simulink model "Rectifier_3"  (R2022a)
settings: Solver=VariableStepAuto  StartTime=0.0  StopTime=2  RelTol=1e-3
model workspace (MAT data in the model file):
  reset = 0
undefined symbols (not defined in the file): DiscIntNeverNeededParam
libraries: spsSeriesRLCBranchLib x38, spsDiodeLib x14, spsCurrentMeasurementLib x12, spsIGBTDiodeLib x8, spsIdealSwitchLib x7, spsMosfetLib x6, spsVoltageMeasurementLib x6, slpidlib x5, spsLinearTransformerLib x4, spsACVoltageSourceLib x3, spsabctodq0Lib x2, simulink x2
settings Model: Creator=zhang  LastModifiedBy=zhang
settings DebuggingCC: UnconnectedInputMsg=warning  UnconnectedOutputMsg=warning  UnconnectedLineMsg=warning
settings RTWCC: DLArmComputeVersion=19.05

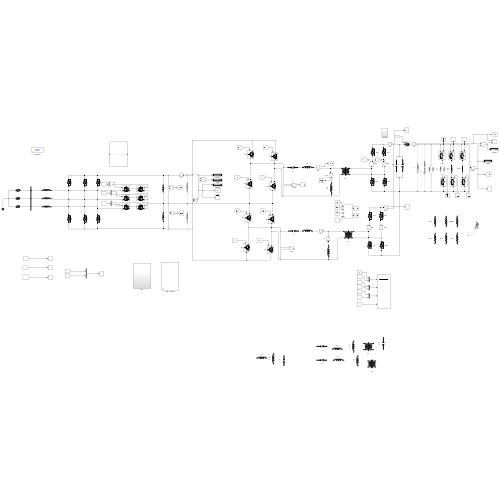
[thumbnail: Simulink's stored preview of the top-level diagram]
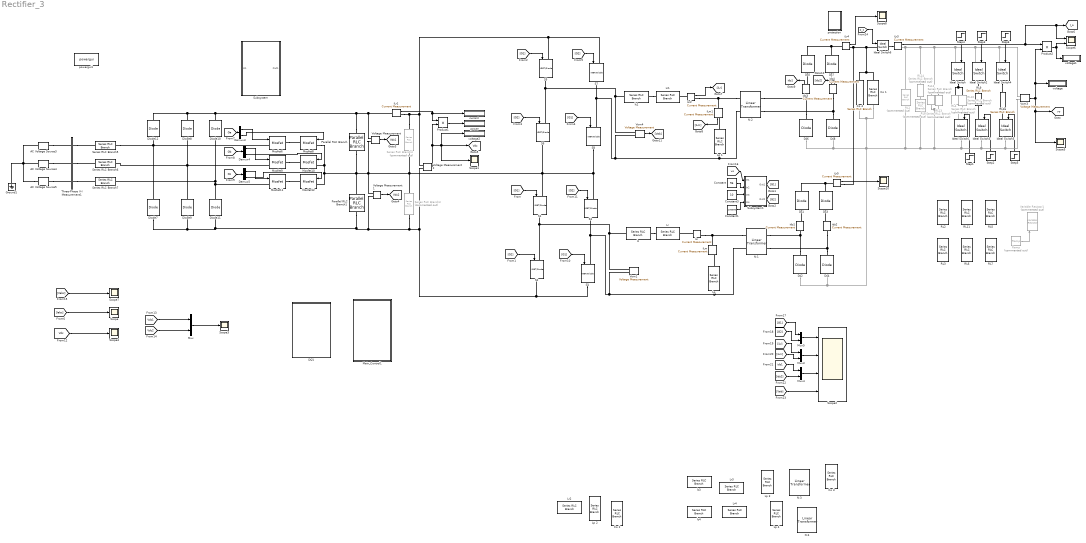
== system Rectifier_3 ==
  " protection" : Subsystem
  AC Voltage Source3 : spsACVoltageSourceLib/AC Voltage Source  Amplitude=311  Phase=0  Frequency=50  SampleTime=0  Measurements=None  BusType=swing  Pref=10e3  Qref=0  Qmin=-inf  Qmax=+inf
  AC Voltage Source4 : spsACVoltageSourceLib/AC Voltage Source  Amplitude=311  Phase=240  Frequency=50  SampleTime=0  Measurements=None  BusType=swing  Pref=10e3  Qref=0  Qmin=-inf  Qmax=+inf
  AC Voltage Source5 : spsACVoltageSourceLib/AC Voltage Source  Amplitude=311  Phase=120  Frequency=50  SampleTime=0  Measurements=None  BusType=swing  Pref=10e3  Qref=0  Qmin=-inf  Qmax=+inf
  Co 1 : spsSeriesRLCBranchLib/Series RLC Branch  LConnTagsString=__new0  RConnTagsString=__new0  BranchType=C  Resistance=1e-3  Inductance=1e-3  SetiL0=off  InitialCurrent=0  Capacitance=10e-3  Setx0=off  InitialVoltage=96  Measurements=None
  Co 2 : spsSeriesRLCBranchLib/Series RLC Branch  LConnTagsString=__new0  RConnTagsString=__new0  BranchType=C  Resistance=1  Inductance=1e-3  SetiL0=off  InitialCurrent=0  Capacitance=660e-6  Setx0=off  InitialVoltage=0  Measurements=None
  Co 3 : spsSeriesRLCBranchLib/Series RLC Branch  LConnTagsString=__new0  RConnTagsString=__new0  BranchType=C  Resistance=1  Inductance=1e-3  SetiL0=off  InitialCurrent=0  Capacitance=2100e-6  Setx0=off  InitialVoltage=0  Measurements=None
  Co 4 : spsSeriesRLCBranchLib/Series RLC Branch  LConnTagsString=__new0  RConnTagsString=__new0  BranchType=C  Resistance=1e-3  Inductance=1e-3  SetiL0=off  InitialCurrent=0  Capacitance=4e-3  Setx0=off  InitialVoltage=96  Measurements=None
  Constant : Constant  Value=96
  Constant1 : Constant  Value=100000
  Constant3 : Constant  Value=10
  DQ1 : Subsystem
  Demux3 : Demux  Outputs=2
  Demux4 : Demux  Outputs=2
  Demux5 : Demux  Outputs=2
  Diode{7..12} (6 alike) : spsDiodeLib/Diode  Ron=0.001  Lon=0  Vf=0.8  IC=0  UseSnubber=off  Rs=1e5  Cs=250e-9  Measurements=off
  Ds{1..8} (8 alike) : spsDiodeLib/Diode  Ron=0.001  Lon=0  Vf=0.8  IC=0  UseSnubber=0  Rs=500  Cs=250e-9  Measurements=off
  Ground1 : spsGroundLib/Ground  LConnTagsString=a
  Ideal Switch{,1..6} (7 alike) : spsIdealSwitchLib/Ideal Switch  Ron=0.001  Lon=0  IC=0  Rs=1e5  Cs=inf  Measurements=off
  "Lp " : spsSeriesRLCBranchLib/Series RLC Branch  LConnTagsString=__new0  RConnTagsString=__new0  BranchType=L  Resistance=1  Inductance=175e-6  SetiL0=off  InitialCurrent=0  Capacitance=1e-6  Setx0=off  InitialVoltage=0  Measurements=None
  Lp 1 : spsSeriesRLCBranchLib/Series RLC Branch  LConnTagsString=__new0  RConnTagsString=__new0  BranchType=L  Resistance=1  Inductance=175e-6  SetiL0=off  InitialCurrent=0  Capacitance=1e-6  Setx0=off  InitialVoltage=0  Measurements=None
  Lp 2 : spsSeriesRLCBranchLib/Series RLC Branch  LConnTagsString=__new0  RConnTagsString=__new0  BranchType=L  Resistance=1  Inductance=180.2e-6  SetiL0=off  InitialCurrent=0  Capacitance=1e-6  Setx0=off  InitialVoltage=0  Measurements=None
  Lp 3 : spsSeriesRLCBranchLib/Series RLC Branch  LConnTagsString=__new0  RConnTagsString=__new0  BranchType=L  Resistance=1  Inductance=79.6e-6  SetiL0=off  InitialCurrent=0  Capacitance=1e-6  Setx0=off  InitialVoltage=0  Measurements=None
  Lp 4 : spsSeriesRLCBranchLib/Series RLC Branch  LConnTagsString=__new0  RConnTagsString=__new0  BranchType=L  Resistance=1  Inductance=66.6e-6  SetiL0=off  InitialCurrent=0  Capacitance=1e-6  Setx0=off  InitialVoltage=0  Measurements=None
  Lr : spsSeriesRLCBranchLib/Series RLC Branch  LConnTagsString=__new0  RConnTagsString=__new0  BranchType=L  Resistance=1  Inductance=36e-6  SetiL0=off  InitialCurrent=0  Capacitance=1e-6  Setx0=off  InitialVoltage=0  Measurements=None
  Lr1 : spsSeriesRLCBranchLib/Series RLC Branch  LConnTagsString=__new0  RConnTagsString=__new0  BranchType=L  Resistance=1  Inductance=36e-6  SetiL0=off  InitialCurrent=0  Capacitance=1e-6  Setx0=off  InitialVoltage=0  Measurements=None
  Lr2 : spsSeriesRLCBranchLib/Series RLC Branch  LConnTagsString=__new0  RConnTagsString=__new0  BranchType=L  Resistance=1  Inductance=20.2e-6  SetiL0=off  InitialCurrent=0  Capacitance=1e-6  Setx0=off  InitialVoltage=0  Measurements=None
  Lr3 : spsSeriesRLCBranchLib/Series RLC Branch  LConnTagsString=__new0  RConnTagsString=__new0  BranchType=L  Resistance=1  Inductance=11.8e-6  SetiL0=off  InitialCurrent=0  Capacitance=1e-6  Setx0=off  InitialVoltage=0  Measurements=None
  Lr4 : spsSeriesRLCBranchLib/Series RLC Branch  LConnTagsString=__new0  RConnTagsString=__new0  BranchType=L  Resistance=1  Inductance=16.8e-6  SetiL0=off  InitialCurrent=0  Capacitance=1e-6  Setx0=off  InitialVoltage=0  Measurements=None
  Main_Control1 : Subsystem  mask{Vref=800, Fs=20000, Kp_v=0.53, Ki_v=0.00025, Kp_i=11, Ki_i=0.3, limit1=40, limit2=450, Kp_vb=0.5, Ki_vb=0.00001, k3=0.245}
      mask prompts: Vref "DC_voltage"; Kp_vb "VoltageBalance_Kp"; Ki_vb "VoltageBalance_Ki"
  Mosfet{6,8..12} (6 alike) : spsMosfetLib/Mosfet  Ron=0.1  Lon=0  Rd=0.01  Vfd=0  IC=0  Rs=1e5  Cs=inf  Measurements=off
  Mux{,3..5} (4 alike) : Mux  Inputs=2
  N:1 : spsLinearTransformerLib/Linear Transformer  UNITS=SI  NominalPower=[ 3e3 20000 ]  winding1=[40 0 0]  winding2=[8 0 0]  ThreeWindings=off  winding3=[355 0 0]  RmLm=[2.3349e+09 0]  Measurements=None  DataType=on
  N:2 : spsLinearTransformerLib/Linear Transformer  UNITS=SI  NominalPower=[ 3e3 20000 ]  winding1=[40 0 0]  winding2=[8 0 0]  ThreeWindings=off  winding3=[355 0 0]  RmLm=[2.3349e+09 0]  Measurements=None  DataType=on
  N:3 : spsLinearTransformerLib/Linear Transformer  UNITS=SI  NominalPower=[ 3e3 20000 ]  winding1=[400 0 0]  winding2=[90 0 0]  ThreeWindings=off  winding3=[355 0 0]  RmLm=[2.3349e+09 0]  Measurements=None  DataType=on
  N:4 : spsLinearTransformerLib/Linear Transformer  UNITS=SI  NominalPower=[ 3e3 20000 ]  winding1=[400 0 0]  winding2=[80 0 0]  ThreeWindings=off  winding3=[355 0 0]  RmLm=[2.3349e+09 0]  Measurements=None  DataType=on
  Parallel RLC Branch : spsParallelRLCBranchLib/Parallel RLC Branch  LConnTagsString=a  RConnTagsString=__new0  BranchType=C  Resistance=51e3  Inductance=1e-3  SetiL0=off  InitialCurrent=0  Capacitance=2e-3  Setx0=on  InitialVoltage=250  Measurements=None
  Parallel RLC Branch1 : spsParallelRLCBranchLib/Parallel RLC Branch  LConnTagsString=a  RConnTagsString=__new0  BranchType=C  Resistance=51e3  Inductance=1e-3  SetiL0=off  InitialCurrent=0  Capacitance=2e-3  Setx0=on  InitialVoltage=250  Measurements=None
  Product1 : Product
  Product2 : Product
  RL{1,4,12,14} (4 alike) : spsSeriesRLCBranchLib/Series RLC Branch  Commented=on  LConnTagsString=__new0  RConnTagsString=__new0  BranchType=R  Resistance=0.9216  Inductance=1e-3  SetiL0=off  InitialCurrent=0  Capacitance=3000e-6  Setx0=off  InitialVoltage=0  Measurements=None
  RL10 : spsSeriesRLCBranchLib/Series RLC Branch  Commented=on  LConnTagsString=__new0  RConnTagsString=__new0  BranchType=C  Resistance=0.9216  Inductance=1e-3  SetiL0=off  InitialCurrent=0  Capacitance=3000e-6  Setx0=off  InitialVoltage=0  Measurements=None
  RL11 : spsSeriesRLCBranchLib/Series RLC Branch  LConnTagsString=__new0  RConnTagsString=__new0  BranchType=R  Resistance=1.2288  Inductance=1e-3  SetiL0=off  InitialCurrent=0  Capacitance=2200e-6  Setx0=off  InitialVoltage=0  Measurements=None
  RL13 : spsSeriesRLCBranchLib/Series RLC Branch  Commented=on  LConnTagsString=__new0  RConnTagsString=__new0  BranchType=C  Resistance=0.9216  Inductance=1e-3  SetiL0=off  InitialCurrent=0  Capacitance=3000e-6  Setx0=off  InitialVoltage=0  Measurements=None
  RL16 : spsSeriesRLCBranchLib/Series RLC Branch  LConnTagsString=__new0  RConnTagsString=__new0  BranchType=R  Resistance=3  Inductance=1e-3  SetiL0=off  InitialCurrent=0  Capacitance=3000e-6  Setx0=off  InitialVoltage=0  Measurements=None
  RL2 : spsSeriesRLCBranchLib/Series RLC Branch  LConnTagsString=__new0  RConnTagsString=__new0  BranchType=R  Resistance=1.8432  Inductance=1e-3  SetiL0=off  InitialCurrent=0  Capacitance=2200e-6  Setx0=off  InitialVoltage=0  Measurements=None
  RL3 : spsSeriesRLCBranchLib/Series RLC Branch  LConnTagsString=__new0  RConnTagsString=__new0  BranchType=R  Resistance=3.6864  Inductance=1e-3  SetiL0=off  InitialCurrent=0  Capacitance=2200e-6  Setx0=off  InitialVoltage=0  Measurements=None
  RL5 : spsSeriesRLCBranchLib/Series RLC Branch  LConnTagsString=__new0  RConnTagsString=__new0  BranchType=R  Resistance=1.8432  Inductance=1e-3  SetiL0=off  InitialCurrent=0  Capacitance=2200e-6  Setx0=off  InitialVoltage=0  Measurements=None
  RL6 : spsSeriesRLCBranchLib/Series RLC Branch  LConnTagsString=__new0  RConnTagsString=__new0  BranchType=R  Resistance=1.8432  Inductance=1e-3  SetiL0=off  InitialCurrent=0  Capacitance=2200e-6  Setx0=off  InitialVoltage=0  Measurements=None
  RL7 : spsSeriesRLCBranchLib/Series RLC Branch  LConnTagsString=__new0  RConnTagsString=__new0  BranchType=R  Resistance=3.6864  Inductance=1e-3  SetiL0=off  InitialCurrent=0  Capacitance=2200e-6  Setx0=off  InitialVoltage=0  Measurements=None
  RL8 : spsSeriesRLCBranchLib/Series RLC Branch  Commented=on  LConnTagsString=__new0  RConnTagsString=__new0  BranchType=C  Resistance=0.9216  Inductance=1e-3  SetiL0=off  InitialCurrent=0  Capacitance=3000e-6  Setx0=off  InitialVoltage=0  Measurements=None
  RL9 : spsSeriesRLCBranchLib/Series RLC Branch  LConnTagsString=__new0  RConnTagsString=__new0  BranchType=R  Resistance=0.9216  Inductance=1e-3  SetiL0=off  InitialCurrent=0  Capacitance=3000e-6  Setx0=off  InitialVoltage=0  Measurements=None
  Ramp : simulink/Sources/Ramp  Commented=on  slope=9600000  start=0  InitialOutput=0
  S{1..8} (8 alike) : spsIGBTDiodeLib/IGBT//Diode  Ron=1e-3  Rs=1e5  Cs=250e-9  Measurements=off
  Scope{,1,3..5,7..8,10} (8 alike) : Scope
  Scope2 : Scope  NumInputPorts=4
  Scope6 : Scope  NumInputPorts=2
  Series RLC Branch3 : spsSeriesRLCBranchLib/Series RLC Branch  Commented=on  LConnTagsString=__new0  RConnTagsString=__new0  BranchType=R  Resistance=32  Inductance=2e-3  SetiL0=off  InitialCurrent=0  Capacitance=1e-6  Setx0=off  InitialVoltage=0  Measurements=None
  Series RLC Branch4 : spsSeriesRLCBranchLib/Series RLC Branch  Commented=on  LConnTagsString=__new0  RConnTagsString=__new0  BranchType=R  Resistance=32  Inductance=2e-3  SetiL0=off  InitialCurrent=0  Capacitance=1e-6  Setx0=off  InitialVoltage=0  Measurements=None
  Series RLC Branch5 : spsSeriesRLCBranchLib/Series RLC Branch  LConnTagsString=__new0  RConnTagsString=__new0  BranchType=L  Resistance=20  Inductance=2.5e-3  SetiL0=off  InitialCurrent=0  Capacitance=1e-6  Setx0=off  InitialVoltage=0  Measurements=None
  Series RLC Branch6 : spsSeriesRLCBranchLib/Series RLC Branch  LConnTagsString=__new0  RConnTagsString=__new0  BranchType=L  Resistance=20  Inductance=2.5e-3  SetiL0=off  InitialCurrent=0  Capacitance=1e-6  Setx0=off  InitialVoltage=0  Measurements=None
  Series RLC Branch7 : spsSeriesRLCBranchLib/Series RLC Branch  LConnTagsString=__new0  RConnTagsString=__new0  BranchType=L  Resistance=20  Inductance=2.5e-3  SetiL0=off  InitialCurrent=0  Capacitance=1e-6  Setx0=off  InitialVoltage=0  Measurements=None
  Step1 : Step  Time=0.4  Before=1  After=0  SampleTime=0
  Step2 : Step  Time=0.5  Before=1  After=0  SampleTime=0
  Step3 : Step  Time=0  SampleTime=0
  Step4 : Step  Time=0.2  SampleTime=0
  Step5 : Step  Time=1.5  Before=1  After=0  SampleTime=0
  Step6 : Step  SampleTime=0
  Subsystem : Subsystem
      settings: OpenFcn="open(\"C:\\Users\\zhang\\Desktop\\仿真\\pros\""
  Subsystem1 : Subsystem  mask{P=35000, I=5000}
      mask DialogControl ParameterGroupVar Prompt: 参数
  Three-Phase V-I Measurement1 : spsThreePhaseVIMeasurementLib/Three-Phase V-I Measurement  VoltageMeasurement=phase-to-ground  SetLabelV=on  LabelV=Vabc  Vpu=off  VpuLL=off  CurrentMeasurement=yes  SetLabelI=on  LabelI=Iabc  Ipu=off  Pbase=100e6  Vbase=500e3  OutputType=Complex  PhasorSimulation=off  PSBequivalent=0
  Variable Resistor1 : spsVariableResistorLib/Variable Resistor  Commented=on  Rabsmin=1.8432
      settings: SourceProductBaseCode=PS
  Voltage Measurement : spsVoltageMeasurementLib/Voltage Measurement  PhasorSimulation=off  OutputType=Complex  PSBequivalent=0
  Voltage Measurement1 : spsVoltageMeasurementLib/Voltage Measurement  PhasorSimulation=off  OutputType=Complex  PSBequivalent=0
  Voltage Measurement2 : spsVoltageMeasurementLib/Voltage Measurement  PhasorSimulation=off  OutputType=Complex  PSBequivalent=0
  Vom1 : spsVoltageMeasurementLib/Voltage Measurement  PhasorSimulation=off  OutputType=Complex  PSBequivalent=0
  Vom3 : spsVoltageMeasurementLib/Voltage Measurement  PhasorSimulation=off  OutputType=Complex  PSBequivalent=0
  Vom4 : spsVoltageMeasurementLib/Voltage Measurement  PhasorSimulation=off  OutputType=Complex  PSBequivalent=0
  current : Display
  iLm : spsCurrentMeasurementLib/Current Measurement  PhasorSimulation=off  OutputType=Complex  PSBequivalent=0
  iLm1 : spsCurrentMeasurementLib/Current Measurement  PhasorSimulation=off  OutputType=Complex  PSBequivalent=0
  iLr{,1..5} (6 alike) : spsCurrentMeasurementLib/Current Measurement  PhasorSimulation=off  OutputType=Complex  PSBequivalent=0
  ids{1..4} (4 alike) : spsCurrentMeasurementLib/Current Measurement  PhasorSimulation=off  OutputType=Complex  PSBequivalent=0
  lc : spsSeriesRLCBranchLib/Series RLC Branch  LConnTagsString=__new0  RConnTagsString=__new0  BranchType=C  Resistance=1  Inductance=1e-3  SetiL0=off  InitialCurrent=0  Capacitance=89.5e-9  Setx0=off  InitialVoltage=0  Measurements=None
  lc1 : spsSeriesRLCBranchLib/Series RLC Branch  LConnTagsString=__new0  RConnTagsString=__new0  BranchType=C  Resistance=1  Inductance=1e-3  SetiL0=off  InitialCurrent=0  Capacitance=89.5e-9  Setx0=off  InitialVoltage=0  Measurements=None
  lc3 : spsSeriesRLCBranchLib/Series RLC Branch  LConnTagsString=__new0  RConnTagsString=__new0  BranchType=C  Resistance=1  Inductance=1e-3  SetiL0=off  InitialCurrent=0  Capacitance=100.4e-9  Setx0=off  InitialVoltage=0  Measurements=None
  lc4 : spsSeriesRLCBranchLib/Series RLC Branch  LConnTagsString=__new0  RConnTagsString=__new0  BranchType=C  Resistance=1  Inductance=1e-3  SetiL0=off  InitialCurrent=0  Capacitance=200.4e-9  Setx0=off  InitialVoltage=0  Measurements=None
  power : Display
  powergui1 : spspowerguiLib/powergui  Priority=1  SimulationMode=Discrete  SampleTime=1e-6  frequency=60  Iterations=50  frequencyindice=0  Pbase=100e6  ErrMax=1e-4  UnitsV=kV  UnitsW=MW  buscounter=0  FunctionMessages=off  echomessages=off  EnableUseOfTLC=off  CurrentSourceSwitches=off  DisableSnubberDevices=off  DisableRonSwitches=off  DisableVfSwitches=off  DisplayEquations=off  AutomaticDiscreteSolvers=off  SolverType=Tustin/Backward Euler (TBE)  Interpol=off  ExternalGateDelay=off  methode=off  Ts=100  x0status=blocks  SPID=on  SwTol=0  HookPort=off  NonlinearTolerance=1e-4  nMaxIteration=100  ContinueOnMaxIteration=off  RestoreLinks=warning  ResistiveCurrentMeasurement=off  Frange=[0:2:500]  Ylog=off  Xlog=on  ShowGrid=off  save=off  variable=ZData  structure=0  ZoomFFT=off  StartTime=0.0  cycles=1  DisplayStyle=1  fundamental=60  FreqAxis=off  MaxFrequency=1000  frequencyindicesteady=1  RmsSteady=1  display=off
  voltage : Display
  voltage1 : Display
  voltage2 : Display
  tag scope: I_o=global, Vdc1=global, Vdc2=global, Vdc=global, ids1=global, vo=global
  wires:
  [G1] -> S4/1
  [G2] -> S3/1
  [G1] -> S1/1
  [G2] -> S2/1
  Product2/1 -> Scope6/2, voltage1/1
  iLr3/1 -> Scope6/1, [I_o], Product2/1
  [G1] -> S8/1
  iLm1/1 -> [iLm]
  ids3/1 -> [ids1]
  iLr2/1 -> [iLr]
  ids4/1 -> [ids2]
  [G2] -> S7/1
  [G1] -> S5/1
  Vom4/1 -> [Vab]
  Vom3/1 -> [vo], Scope5/1, Product2/2, voltage/1
  [G2] -> S6/1
  [iLm] -> Mux3/2
  Constant/1 -> Subsystem1/2(In2)
  Subsystem1/1(Out1) -> [G1]
  Subsystem1/2(Out2) -> [G2]
  Constant3/1 -> Subsystem1/3(In3)
  Constant1/1 -> Subsystem1/4(In4)
  [ids1] -> Mux4/1
  [vo] -> Subsystem1/1(In1)
  Mux4/1 -> Scope2/3
  [ids2] -> Mux4/2
  Mux3/1 -> Scope2/2
  Mux5/1 -> Scope2/1
  [G2] -> Mux5/2
  [Vab] -> Scope2/4
  [G1] -> Mux5/1
  [iLr] -> Mux3/1
  Step1/1 -> Ideal Switch1/1
  Step4/1 -> Ideal Switch/1
  Step3/1 -> Ideal Switch2/1
  Step2/1 -> Ideal Switch3/1
  Step5/1 -> Ideal Switch5/1
  Step6/1 -> Ideal Switch4/1
  [o_c] -> Ideal Switch6/1
  iLr5/1 -> Scope10/1
  iLr4/1 -> Scope8/1
  Ramp/1 -> Variable Resistor1/1
  Voltage Measurement2/1 -> Product1/2, Scope1/1, [Vdc], voltage2/1
  Voltage Measurement/1 -> [Vdc1]
  Demux3/1 -> Mosfet6/1
  Demux5/2 -> Mosfet12/1
  Product1/1 -> power/1
  Demux3/2 -> Mosfet8/1
  Demux4/1 -> Mosfet9/1
  [Gb] -> Demux4/1
  [Ga] -> Demux3/1
  Demux4/2 -> Mosfet10/1
  iLr1/1 -> Product1/1, current/1
  Demux5/1 -> Mosfet11/1
  Voltage Measurement1/1 -> [Vdc2]
  [Gc] -> Demux5/1
  Mux/1 -> Scope3/1
  [Vdc1] -> Mux/1
  [Vdc2] -> Mux/2
  [Vdc] -> Scope4/1
  [Iabc] -> Scope/1
  [Vabc] -> Scope7/1
  connections:
  S3/RConn1 -- S4/LConn1 -- "Lp "/RConn1 -- N:1/LConn2 -- Vom1/LConn2
  Ds2/RConn1 -- ids1/LConn1 -- N:1/RConn1
  N:1/LConn1 -- iLr/RConn1 -- iLm/LConn1
  Ds4/RConn1 -- ids2/LConn1 -- N:1/RConn2
  S2/LConn1 -- S1/RConn1 -- Vom1/LConn1 -- lc/LConn1
  iLr/LConn1 -- Lr/LConn1
  ids2/RConn1 -- Ds3/LConn1
  "Lp "/LConn1 -- iLm/RConn1
  lc/RConn1 -- Lr/RConn1
  ids1/RConn1 -- Ds1/LConn1
  S7/RConn1 -- S8/LConn1 -- Lp 1/RConn1 -- N:2/LConn2 -- Vom4/LConn2
  Ds6/RConn1 -- ids3/LConn1 -- N:2/RConn1
  N:2/LConn1 -- iLr2/RConn1 -- iLm1/LConn1
  Ds8/RConn1 -- ids4/LConn1 -- N:2/RConn2
  S6/LConn1 -- S5/RConn1 -- Vom4/LConn1 -- lc1/LConn1
  iLr2/LConn1 -- Lr1/LConn1
  ids4/RConn1 -- Ds7/LConn1
  Lp 1/LConn1 -- iLm1/RConn1
  ids3/RConn1 -- Ds5/LConn1
  RL13/LConn1 -- RL14/LConn1 -- RL1/LConn1 -- iLr3/RConn1 -- Vom3/LConn1 -- Ideal Switch4/LConn1 -- Ideal Switch2/LConn1 -- Ideal Switch/LConn1 -- RL12/LConn1
  RL12/RConn1 -- RL13/RConn1 -- Ds4/LConn1 -- Ds2/LConn1 -- Co 1/RConn1 -- Co 4/RConn1 -- Ds6/LConn1 -- Ds8/LConn1 -- RL1/RConn1 -- RL8/RConn1 -- Ideal Switch5/RConn1 -- Vom3/LConn2 -- Ideal Switch3/RConn1 -- Ideal Switch1/RConn1
  Ds7/RConn1 -- iLr4/LConn1 -- Ds5/RConn1
  Co 1/LConn1 -- iLr5/RConn1 -- iLr4/RConn1 -- Ideal Switch6/LConn1 -- Co 4/LConn1
  Ideal Switch3/LConn1 -- RL9/RConn1
  Ds3/RConn1 -- Ds1/RConn1 -- iLr5/LConn1
  lc1/RConn1 -- Lr1/RConn1
  RL14/RConn1 -- RL8/LConn1
  Ideal Switch5/LConn1 -- RL16/RConn1
  Voltage Measurement1/LConn2 -- Diode7/LConn1 -- Diode9/LConn1 -- Diode11/LConn1 -- Parallel RLC Branch1/RConn1 -- Voltage Measurement2/LConn2 -- S4/RConn1 -- S2/RConn1 -- Series RLC Branch3/RConn1
  Series RLC Branch4/LConn1 -- Voltage Measurement2/LConn1 -- S7/LConn1 -- S5/LConn1 -- iLr1/RConn1
  Ideal Switch4/RConn1 -- RL16/LConn1
  Mosfet10/LConn1 -- Mosfet8/LConn1 -- Series RLC Branch4/RConn1 -- S6/RConn1 -- S3/LConn1 -- S8/RConn1 -- S1/LConn1 -- Series RLC Branch3/LConn1 -- Voltage Measurement/LConn2 -- Voltage Measurement1/LConn1 -- Parallel RLC Branch/RConn1 -- Parallel RLC Branch1/LConn1 -- Mosfet12/LConn1
  Parallel RLC Branch/LConn1 -- Diode12/RConn1 -- Diode8/RConn1 -- Diode10/RConn1 -- Voltage Measurement/LConn1 -- iLr1/LConn1
  Diode11/RConn1 -- Mosfet11/LConn1 -- Diode10/LConn1 -- Series RLC Branch7/RConn1
  Diode8/LConn1 -- Diode9/RConn1 -- Mosfet9/LConn1 -- Series RLC Branch6/RConn1
  Series RLC Branch5/RConn1 -- Diode7/RConn1 -- Diode12/LConn1 -- Mosfet6/LConn1
  AC Voltage Source5/LConn1 -- AC Voltage Source4/LConn1 -- AC Voltage Source3/LConn1 -- Ground1/LConn1
  Three-Phase V-I Measurement1/RConn2 -- Series RLC Branch6/LConn1
  Three-Phase V-I Measurement1/RConn1 -- Series RLC Branch5/LConn1
  Mosfet9/RConn1 -- Mosfet10/RConn1
  AC Voltage Source3/RConn1 -- Three-Phase V-I Measurement1/LConn1
  Mosfet11/RConn1 -- Mosfet12/RConn1
  Mosfet6/RConn1 -- Mosfet8/RConn1
  AC Voltage Source4/RConn1 -- Three-Phase V-I Measurement1/LConn2
  AC Voltage Source5/RConn1 -- Three-Phase V-I Measurement1/LConn3
  Three-Phase V-I Measurement1/RConn3 -- Series RLC Branch7/LConn1
  RL4/RConn1 -- RL10/RConn1 -- Ideal Switch1/LConn1
  Ideal Switch/RConn1 -- RL10/LConn1 -- RL4/LConn1
  RL9/LConn1 -- Ideal Switch2/RConn1
  Ideal Switch6/RConn1 -- iLr3/LConn1

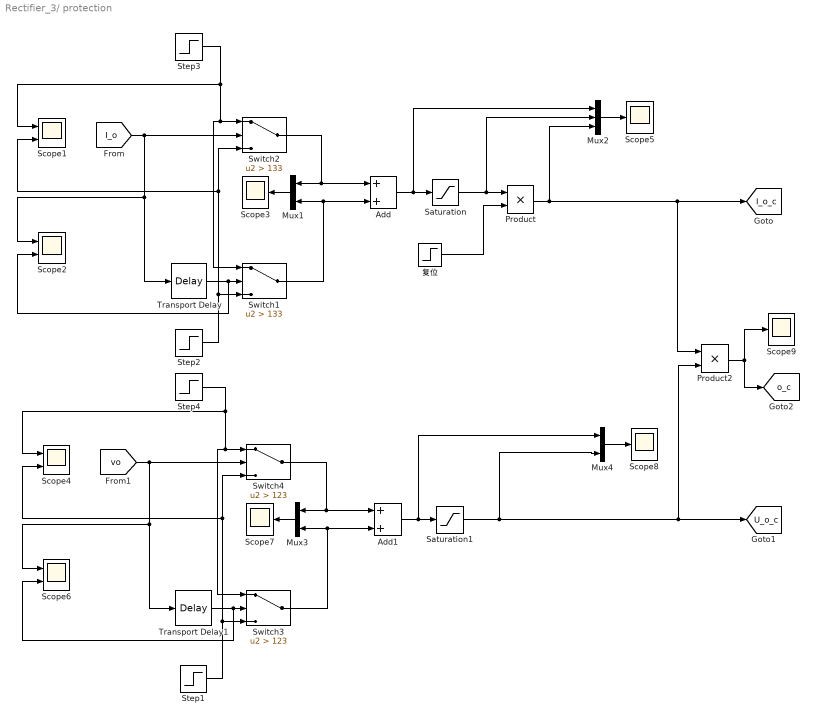
== system Rectifier_3/ protection ==
  Add : Sum
  Add1 : Sum
  Mux1 : Mux  Inputs=2
  Mux2 : Mux  Inputs=3
  Mux3 : Mux  Inputs=2
  Mux4 : Mux  Inputs=2
  Product : Product
  Product2 : Product
  Saturation : Saturate  UpperLimit=1  LowerLimit=0
  Saturation1 : Saturate  UpperLimit=1  LowerLimit=0
  Scope{1..2,4,6} (4 alike) : Scope  NumInputPorts=2
  Scope{3,5,7..9} (5 alike) : Scope
  Step1 : Step  Time=0  Before=1  SampleTime=0
  Step2 : Step  Time=0  Before=1  SampleTime=0
  Step3 : Step  Time=0  After=0  SampleTime=0
  Step4 : Step  Time=0  After=0  SampleTime=0
  Switch1 : Switch  Criteria=u2 > Threshold  Threshold=133  ZeroCross=off  SaturateOnIntegerOverflow=off  InputSameDT=off
  Switch2 : Switch  Criteria=u2 > Threshold  Threshold=133  ZeroCross=off  SaturateOnIntegerOverflow=off  InputSameDT=off
  Switch3 : Switch  Criteria=u2 > Threshold  Threshold=123  ZeroCross=off  SaturateOnIntegerOverflow=off  InputSameDT=off
  Switch4 : Switch  Criteria=u2 > Threshold  Threshold=123  ZeroCross=off  SaturateOnIntegerOverflow=off  InputSameDT=off
  Transport Delay : TransportDelay  DelayTime=0.05
  Transport Delay1 : TransportDelay  DelayTime=0.05
  复位 : Step  Time=0  Before=1  SampleTime=0
  tag scope: I_o_c=global, U_o_c=global, o_c=global
  wires:
  Switch2/1 -> Mux1/1, Add/1
  Step3/1 -> Switch1/1, Switch2/1, Scope1/1
  Step2/1 -> Scope1/2, Switch2/3, Switch1/3
  [I_o] -> Switch2/2, Scope2/1, Transport Delay/1
  Transport Delay/1 -> Scope2/2, Switch1/2
  Switch1/1 -> Mux1/2, Add/2
  Add/1 -> Mux2/1, Saturation/1
  Saturation/1 -> Product/1, Mux2/2
  Mux1/1 -> Scope3/1
  Product/1 -> Mux2/3, [I_o_c], Product2/1
  复位/1 -> Product/2
  Mux2/1 -> Scope5/1
  Saturation1/1 -> [U_o_c], Product2/2, Mux4/2
  Mux4/1 -> Scope8/1
  Mux3/1 -> Scope7/1
  Transport Delay1/1 -> Scope6/2, Switch3/2
  Add1/1 -> Mux4/1, Saturation1/1
  [vo] -> Switch4/2, Scope6/1, Transport Delay1/1
  Step1/1 -> Scope4/2, Switch4/3, Switch3/3
  Step4/1 -> Switch3/1, Switch4/1, Scope4/1
  Switch4/1 -> Mux3/1, Add1/1
  Switch3/1 -> Mux3/2, Add1/2
  Product2/1 -> Scope9/1, [o_c]

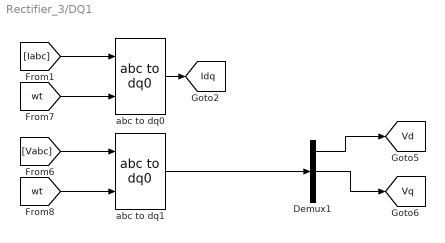
== system Rectifier_3/DQ1 ==
  Demux1 : Demux  Outputs=3
  abc to dq0 : spsabctodq0Lib/abc to dq0  Alignment=90 degrees behind phase A axis
  abc to dq1 : spsabctodq0Lib/abc to dq0  Alignment=90 degrees behind phase A axis
  tag scope: Idq=global, Vd=global, Vq=global
  wires:
  [Iabc] -> abc to dq0/1
  abc to dq0/1 -> [Idq]
  [Vabc] -> abc to dq1/1
  Demux1/2 -> [Vq]
  Demux1/1 -> [Vd]
  abc to dq1/1 -> Demux1/1
  [wt] -> abc to dq0/2
  [wt] -> abc to dq1/2

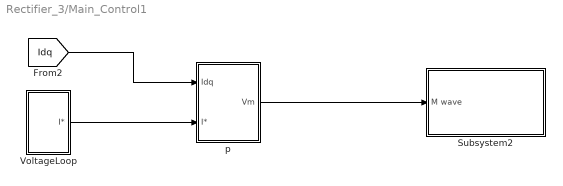
== system Rectifier_3/Main_Control1 ==
  Subsystem2 : Subsystem
  VoltageLoop : Subsystem
  p : Subsystem
  wires:
  [Idq] -> p/1(Idq)
  p/1(Vm) -> Subsystem2/1(M wave)
  VoltageLoop/1(I*) -> p/2(I*)

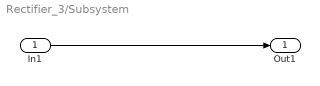
== system Rectifier_3/Subsystem ==
  In1 : Inport
  Out1 : Outport
  wires:
  In1/1 -> Out1/1

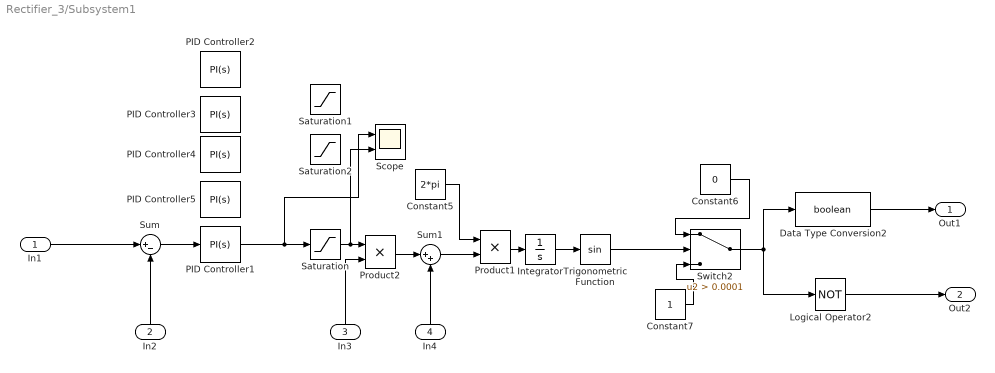
== system Rectifier_3/Subsystem1 ==
  In1 : Inport
  In2 : Inport  Port=2
  In3 : Inport  Port=3
  In4 : Inport  Port=4
  Constant5 : Constant  Value=2*pi
  Constant6 : Constant  Value=0
  Constant7 : Constant
  Data Type Conversion2 : DataTypeConversion  OutDataTypeStr=boolean  SaturateOnIntegerOverflow=off  RndMeth=Floor
  Integrator : Integrator
  Logical Operator2 : Logic  Operator=NOT  AllPortsSameDT=off  OutDataTypeStr=boolean
  PID Controller1 : slpidlib/PID Controller  Controller=PI  Form=Parallel  TimeDomain=Continuous-time  UseExternalTs=off  SampleTime=-1  IntegratorMethod=Forward Euler  FilterMethod=Forward Euler  ControllerParametersSource=internal  P=P  I=I  UseKiTs=off  D=3  N=100  UseFilter=on  TunerSelectOption=Transfer Function Based (PID Tuner App)  InitialConditionSource=internal  InitialConditionForIntegrator=0  InitialConditionForFilter=0  DifferentiatorICPrevScaledInput=0  ExternalReset=none  TrackingMode=off  Kt=1  LimitOutput=off  SatLimitsSource=internal  UpperSaturationLimit=inf  LowerSaturationLimit=-inf  LinearizeAsGain=on  AntiWindupMode=none  Kb=1  POutMin=[]  POutMax=[]  IOutMin=[]  IOutMax=[]  DOutMin=[]  DOutMax=[]  NOutMin=[]  NOutMax=[]  SumOutMin=[]  SumOutMax=[]  SaturationOutMin=[]  SaturationOutMax=[]  PParamMin=[]  PParamMax=[]  IParamMin=[]  IParamMax=[]  DParamMin=[]  DParamMax=[]  NParamMin=[]  NParamMax=[]  KbParamMin=[]  KbParamMax=[]  KtParamMin=[]  KtParamMax=[]  KbOutMin=[]  KbOutMax=[]  KtOutMin=[]  KtOutMax=[]  IntegratorOutMin=[]  IntegratorOutMax=[]  FilterOutMin=[]  FilterOutMax=[]  SumI1OutMin=[]  SumI1OutMax=[]  SumI2OutMin=[]  SumI2OutMax=[]  SumI3OutMin=[]  SumI3OutMax=[]  SumI4OutMin=[]  SumI4OutMax=[]  SumDOutMin=[]  SumDOutMax=[]  DifferentiatorOutMin=[]  DifferentiatorOutMax=[]  FilterDiffOutCoefMin=[]  FilterDiffOutCoefMax=[]  ReciprocalOutMin=[]  ReciprocalOutMax=[]  SumDenOutMin=[]  SumDenOutMax=[]  SumNumOutMin=[]  SumNumOutMax=[]  DivideOutMin=[]  DivideOutMax=[]  UdiffTsProdOutMin=[]  UdiffTsProdOutMax=[]  NTsProdOutMin=[]  NTsProdOutMax=[]  UintegralTsProdOutMin=[]  UintegralTsProdOutMax=[]  UngainTsProdOutMin=[]  UngainTsProdOutMax=[]  IntegratorContinuousStateAttributes=''  IntegratorStateMustResolveToSignalObject=off  IntegratorRTWStateStorageClass=Auto  FilterContinuousStateAttributes=''  FilterStateMustResolveToSignalObject=off  FilterRTWStateStorageClass=Auto  ParallelPVariant=InternalParameters  IdealPVariant=Disabled  IVariant=InternalParameters  DVariant=Disabled  IntegratorVariant=Continuous  SatVariant=Disabled  AWVariant=Passthrough  PCopyVariant=Disabled  TRVariant=Disabled  FdbkBlocksVariant=Forward  IdealPFdbkVariant=Disabled  SatFdbkVariant=Disabled  DerivativeFilterVariant=Disabled  NVariant=Disabled  NCopyVariant=Disabled_SignalSpec  FilterICVariant=Disabled  IntegratorICVariant=InternalICs  ExternalResetVariant=Disabled  TRSumVariant=Passthrough  SumFdbkVariant=Disabled  SumVariant=Sum_PI  TsampFilterVariant=InternalTs  TsampNgainVariant=Passthrough  TsampIntegralVariant=Passthrough  ExternalSaturationOutDataTypeStr=Inherit: Same as second input  aMode=0
  PID Controller2 : slpidlib/PID Controller  Controller=PI  Form=Parallel  TimeDomain=Continuous-time  UseExternalTs=off  SampleTime=-1  IntegratorMethod=Forward Euler  FilterMethod=Forward Euler  ControllerParametersSource=internal  P=500  I=35000  UseKiTs=off  D=0  N=100  UseFilter=on  TunerSelectOption=Transfer Function Based (PID Tuner App)  InitialConditionSource=internal  InitialConditionForIntegrator=0  InitialConditionForFilter=0  DifferentiatorICPrevScaledInput=0  ExternalReset=none  TrackingMode=off  Kt=1  LimitOutput=off  SatLimitsSource=internal  UpperSaturationLimit=inf  LowerSaturationLimit=-inf  LinearizeAsGain=on  AntiWindupMode=none  Kb=1  POutMin=[]  POutMax=[]  IOutMin=[]  IOutMax=[]  DOutMin=[]  DOutMax=[]  NOutMin=[]  NOutMax=[]  SumOutMin=[]  SumOutMax=[]  SaturationOutMin=[]  SaturationOutMax=[]  PParamMin=[]  PParamMax=[]  IParamMin=[]  IParamMax=[]  DParamMin=[]  DParamMax=[]  NParamMin=[]  NParamMax=[]  KbParamMin=[]  KbParamMax=[]  KtParamMin=[]  KtParamMax=[]  KbOutMin=[]  KbOutMax=[]  KtOutMin=[]  KtOutMax=[]  IntegratorOutMin=[]  IntegratorOutMax=[]  FilterOutMin=[]  FilterOutMax=[]  SumI1OutMin=[]  SumI1OutMax=[]  SumI2OutMin=[]  SumI2OutMax=[]  SumI3OutMin=[]  SumI3OutMax=[]  SumI4OutMin=[]  SumI4OutMax=[]  SumDOutMin=[]  SumDOutMax=[]  DifferentiatorOutMin=[]  DifferentiatorOutMax=[]  FilterDiffOutCoefMin=[]  FilterDiffOutCoefMax=[]  ReciprocalOutMin=[]  ReciprocalOutMax=[]  SumDenOutMin=[]  SumDenOutMax=[]  SumNumOutMin=[]  SumNumOutMax=[]  DivideOutMin=[]  DivideOutMax=[]  UdiffTsProdOutMin=[]  UdiffTsProdOutMax=[]  NTsProdOutMin=[]  NTsProdOutMax=[]  UintegralTsProdOutMin=[]  UintegralTsProdOutMax=[]  UngainTsProdOutMin=[]  UngainTsProdOutMax=[]  IntegratorContinuousStateAttributes=''  IntegratorStateMustResolveToSignalObject=off  IntegratorRTWStateStorageClass=Auto  FilterContinuousStateAttributes=''  FilterStateMustResolveToSignalObject=off  FilterRTWStateStorageClass=Auto  ParallelPVariant=InternalParameters  IdealPVariant=Disabled  IVariant=InternalParameters  DVariant=Disabled  IntegratorVariant=Continuous  SatVariant=Disabled  AWVariant=Passthrough  PCopyVariant=Disabled  TRVariant=Disabled  FdbkBlocksVariant=Forward  IdealPFdbkVariant=Disabled  SatFdbkVariant=Disabled  DerivativeFilterVariant=Disabled  NVariant=Disabled  NCopyVariant=Disabled_SignalSpec  FilterICVariant=Disabled  IntegratorICVariant=InternalICs  ExternalResetVariant=Disabled  TRSumVariant=Passthrough  SumFdbkVariant=Disabled  SumVariant=Sum_PI  TsampFilterVariant=InternalTs  TsampNgainVariant=Passthrough  TsampIntegralVariant=Passthrough  ExternalSaturationOutDataTypeStr=Inherit: Same as second input  aMode=0
  PID Controller3 : slpidlib/PID Controller  Controller=PI  Form=Parallel  TimeDomain=Continuous-time  UseExternalTs=off  SampleTime=-1  IntegratorMethod=Forward Euler  FilterMethod=Forward Euler  ControllerParametersSource=internal  P=1400  I=45000  UseKiTs=off  D=0  N=100  UseFilter=on  TunerSelectOption=Transfer Function Based (PID Tuner App)  InitialConditionSource=internal  InitialConditionForIntegrator=0  InitialConditionForFilter=0  DifferentiatorICPrevScaledInput=0  ExternalReset=none  TrackingMode=off  Kt=1  LimitOutput=off  SatLimitsSource=internal  UpperSaturationLimit=inf  LowerSaturationLimit=-inf  LinearizeAsGain=on  AntiWindupMode=none  Kb=1  POutMin=[]  POutMax=[]  IOutMin=[]  IOutMax=[]  DOutMin=[]  DOutMax=[]  NOutMin=[]  NOutMax=[]  SumOutMin=[]  SumOutMax=[]  SaturationOutMin=[]  SaturationOutMax=[]  PParamMin=[]  PParamMax=[]  IParamMin=[]  IParamMax=[]  DParamMin=[]  DParamMax=[]  NParamMin=[]  NParamMax=[]  KbParamMin=[]  KbParamMax=[]  KtParamMin=[]  KtParamMax=[]  KbOutMin=[]  KbOutMax=[]  KtOutMin=[]  KtOutMax=[]  IntegratorOutMin=[]  IntegratorOutMax=[]  FilterOutMin=[]  FilterOutMax=[]  SumI1OutMin=[]  SumI1OutMax=[]  SumI2OutMin=[]  SumI2OutMax=[]  SumI3OutMin=[]  SumI3OutMax=[]  SumI4OutMin=[]  SumI4OutMax=[]  SumDOutMin=[]  SumDOutMax=[]  DifferentiatorOutMin=[]  DifferentiatorOutMax=[]  FilterDiffOutCoefMin=[]  FilterDiffOutCoefMax=[]  ReciprocalOutMin=[]  ReciprocalOutMax=[]  SumDenOutMin=[]  SumDenOutMax=[]  SumNumOutMin=[]  SumNumOutMax=[]  DivideOutMin=[]  DivideOutMax=[]  UdiffTsProdOutMin=[]  UdiffTsProdOutMax=[]  NTsProdOutMin=[]  NTsProdOutMax=[]  UintegralTsProdOutMin=[]  UintegralTsProdOutMax=[]  UngainTsProdOutMin=[]  UngainTsProdOutMax=[]  IntegratorContinuousStateAttributes=''  IntegratorStateMustResolveToSignalObject=off  IntegratorRTWStateStorageClass=Auto  FilterContinuousStateAttributes=''  FilterStateMustResolveToSignalObject=off  FilterRTWStateStorageClass=Auto  ParallelPVariant=InternalParameters  IdealPVariant=Disabled  IVariant=InternalParameters  DVariant=Disabled  IntegratorVariant=Continuous  SatVariant=Disabled  AWVariant=Passthrough  PCopyVariant=Disabled  TRVariant=Disabled  FdbkBlocksVariant=Forward  IdealPFdbkVariant=Disabled  SatFdbkVariant=Disabled  DerivativeFilterVariant=Disabled  NVariant=Disabled  NCopyVariant=Disabled_SignalSpec  FilterICVariant=Disabled  IntegratorICVariant=InternalICs  ExternalResetVariant=Disabled  TRSumVariant=Passthrough  SumFdbkVariant=Disabled  SumVariant=Sum_PI  TsampFilterVariant=InternalTs  TsampNgainVariant=Passthrough  TsampIntegralVariant=Passthrough  ExternalSaturationOutDataTypeStr=Inherit: Same as second input  aMode=0
  PID Controller4 : slpidlib/PID Controller  Controller=PI  Form=Parallel  TimeDomain=Continuous-time  UseExternalTs=off  SampleTime=-1  IntegratorMethod=Forward Euler  FilterMethod=Forward Euler  ControllerParametersSource=internal  P=5000  I=20000  UseKiTs=off  D=0  N=100  UseFilter=on  TunerSelectOption=Transfer Function Based (PID Tuner App)  InitialConditionSource=internal  InitialConditionForIntegrator=0  InitialConditionForFilter=0  DifferentiatorICPrevScaledInput=0  ExternalReset=none  TrackingMode=off  Kt=1  LimitOutput=off  SatLimitsSource=internal  UpperSaturationLimit=inf  LowerSaturationLimit=-inf  LinearizeAsGain=on  AntiWindupMode=none  Kb=1  POutMin=[]  POutMax=[]  IOutMin=[]  IOutMax=[]  DOutMin=[]  DOutMax=[]  NOutMin=[]  NOutMax=[]  SumOutMin=[]  SumOutMax=[]  SaturationOutMin=[]  SaturationOutMax=[]  PParamMin=[]  PParamMax=[]  IParamMin=[]  IParamMax=[]  DParamMin=[]  DParamMax=[]  NParamMin=[]  NParamMax=[]  KbParamMin=[]  KbParamMax=[]  KtParamMin=[]  KtParamMax=[]  KbOutMin=[]  KbOutMax=[]  KtOutMin=[]  KtOutMax=[]  IntegratorOutMin=[]  IntegratorOutMax=[]  FilterOutMin=[]  FilterOutMax=[]  SumI1OutMin=[]  SumI1OutMax=[]  SumI2OutMin=[]  SumI2OutMax=[]  SumI3OutMin=[]  SumI3OutMax=[]  SumI4OutMin=[]  SumI4OutMax=[]  SumDOutMin=[]  SumDOutMax=[]  DifferentiatorOutMin=[]  DifferentiatorOutMax=[]  FilterDiffOutCoefMin=[]  FilterDiffOutCoefMax=[]  ReciprocalOutMin=[]  ReciprocalOutMax=[]  SumDenOutMin=[]  SumDenOutMax=[]  SumNumOutMin=[]  SumNumOutMax=[]  DivideOutMin=[]  DivideOutMax=[]  UdiffTsProdOutMin=[]  UdiffTsProdOutMax=[]  NTsProdOutMin=[]  NTsProdOutMax=[]  UintegralTsProdOutMin=[]  UintegralTsProdOutMax=[]  UngainTsProdOutMin=[]  UngainTsProdOutMax=[]  IntegratorContinuousStateAttributes=''  IntegratorStateMustResolveToSignalObject=off  IntegratorRTWStateStorageClass=Auto  FilterContinuousStateAttributes=''  FilterStateMustResolveToSignalObject=off  FilterRTWStateStorageClass=Auto  ParallelPVariant=InternalParameters  IdealPVariant=Disabled  IVariant=InternalParameters  DVariant=Disabled  IntegratorVariant=Continuous  SatVariant=Disabled  AWVariant=Passthrough  PCopyVariant=Disabled  TRVariant=Disabled  FdbkBlocksVariant=Forward  IdealPFdbkVariant=Disabled  SatFdbkVariant=Disabled  DerivativeFilterVariant=Disabled  NVariant=Disabled  NCopyVariant=Disabled_SignalSpec  FilterICVariant=Disabled  IntegratorICVariant=InternalICs  ExternalResetVariant=Disabled  TRSumVariant=Passthrough  SumFdbkVariant=Disabled  SumVariant=Sum_PI  TsampFilterVariant=InternalTs  TsampNgainVariant=Passthrough  TsampIntegralVariant=Passthrough  ExternalSaturationOutDataTypeStr=Inherit: Same as second input  aMode=0
  PID Controller5 : slpidlib/PID Controller  Controller=PI  Form=Parallel  TimeDomain=Continuous-time  UseExternalTs=off  SampleTime=-1  IntegratorMethod=Forward Euler  FilterMethod=Forward Euler  ControllerParametersSource=internal  P=3150  I=13200  UseKiTs=off  D=3  N=100  UseFilter=on  TunerSelectOption=Transfer Function Based (PID Tuner App)  InitialConditionSource=internal  InitialConditionForIntegrator=0  InitialConditionForFilter=0  DifferentiatorICPrevScaledInput=0  ExternalReset=none  TrackingMode=off  Kt=1  LimitOutput=off  SatLimitsSource=internal  UpperSaturationLimit=inf  LowerSaturationLimit=-inf  LinearizeAsGain=on  AntiWindupMode=none  Kb=1  POutMin=[]  POutMax=[]  IOutMin=[]  IOutMax=[]  DOutMin=[]  DOutMax=[]  NOutMin=[]  NOutMax=[]  SumOutMin=[]  SumOutMax=[]  SaturationOutMin=[]  SaturationOutMax=[]  PParamMin=[]  PParamMax=[]  IParamMin=[]  IParamMax=[]  DParamMin=[]  DParamMax=[]  NParamMin=[]  NParamMax=[]  KbParamMin=[]  KbParamMax=[]  KtParamMin=[]  KtParamMax=[]  KbOutMin=[]  KbOutMax=[]  KtOutMin=[]  KtOutMax=[]  IntegratorOutMin=[]  IntegratorOutMax=[]  FilterOutMin=[]  FilterOutMax=[]  SumI1OutMin=[]  SumI1OutMax=[]  SumI2OutMin=[]  SumI2OutMax=[]  SumI3OutMin=[]  SumI3OutMax=[]  SumI4OutMin=[]  SumI4OutMax=[]  SumDOutMin=[]  SumDOutMax=[]  DifferentiatorOutMin=[]  DifferentiatorOutMax=[]  FilterDiffOutCoefMin=[]  FilterDiffOutCoefMax=[]  ReciprocalOutMin=[]  ReciprocalOutMax=[]  SumDenOutMin=[]  SumDenOutMax=[]  SumNumOutMin=[]  SumNumOutMax=[]  DivideOutMin=[]  DivideOutMax=[]  UdiffTsProdOutMin=[]  UdiffTsProdOutMax=[]  NTsProdOutMin=[]  NTsProdOutMax=[]  UintegralTsProdOutMin=[]  UintegralTsProdOutMax=[]  UngainTsProdOutMin=[]  UngainTsProdOutMax=[]  IntegratorContinuousStateAttributes=''  IntegratorStateMustResolveToSignalObject=off  IntegratorRTWStateStorageClass=Auto  FilterContinuousStateAttributes=''  FilterStateMustResolveToSignalObject=off  FilterRTWStateStorageClass=Auto  ParallelPVariant=InternalParameters  IdealPVariant=Disabled  IVariant=InternalParameters  DVariant=Disabled  IntegratorVariant=Continuous  SatVariant=Disabled  AWVariant=Passthrough  PCopyVariant=Disabled  TRVariant=Disabled  FdbkBlocksVariant=Forward  IdealPFdbkVariant=Disabled  SatFdbkVariant=Disabled  DerivativeFilterVariant=Disabled  NVariant=Disabled  NCopyVariant=Disabled_SignalSpec  FilterICVariant=Disabled  IntegratorICVariant=InternalICs  ExternalResetVariant=Disabled  TRSumVariant=Passthrough  SumFdbkVariant=Disabled  SumVariant=Sum_PI  TsampFilterVariant=InternalTs  TsampNgainVariant=Passthrough  TsampIntegralVariant=Passthrough  ExternalSaturationOutDataTypeStr=Inherit: Same as second input  aMode=0
  Product1 : Product
  Product2 : Product
  Saturation : Saturate  UpperLimit=10  LowerLimit=-4800
  Saturation1 : Saturate  UpperLimit=6000  LowerLimit=-3000
  Saturation2 : Saturate  UpperLimit=3750  LowerLimit=-3600
  Scope : Scope  NumInputPorts=2
  Sum : Sum  Inputs=|+-
  Sum1 : Sum  Inputs=|++
  Switch2 : Switch  Criteria=u2 > Threshold  Threshold=0.0001  ZeroCross=off  SaturateOnIntegerOverflow=off  InputSameDT=off
  Trigonometric Function : Trigonometry
  Out1 : Outport
  Out2 : Outport  Port=2
  wires:
  In4/1 -> Sum1/2
  Sum1/1 -> Product1/2
  Product2/1 -> Sum1/1
  Saturation/1 -> Scope/2, Product2/1
  In3/1 -> Product2/2
  Constant5/1 -> Product1/1
  In2/1 -> Sum/2
  Constant6/1 -> Switch2/1
  Switch2/1 -> Logical Operator2/1, Data Type Conversion2/1
  Trigonometric Function/1 -> Switch2/2
  Sum/1 -> PID Controller1/1
  In1/1 -> Sum/1
  Data Type Conversion2/1 -> Out1/1
  Logical Operator2/1 -> Out2/1
  Constant7/1 -> Switch2/3
  Product1/1 -> Integrator/1
  Integrator/1 -> Trigonometric Function/1
  PID Controller1/1 -> Scope/1, Saturation/1

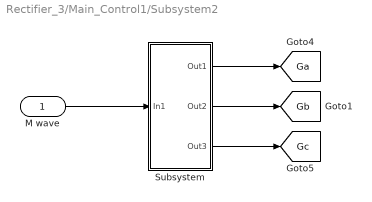
== system Rectifier_3/Main_Control1/Subsystem2 ==
  M wave : Inport
  Subsystem : Subsystem
  tag scope: Ga=global, Gb=global, Gc=global
  wires:
  M wave/1 -> Subsystem/1(In1)
  Subsystem/1(Out1) -> [Ga]
  Subsystem/2(Out2) -> [Gb]
  Subsystem/3(Out3) -> [Gc]

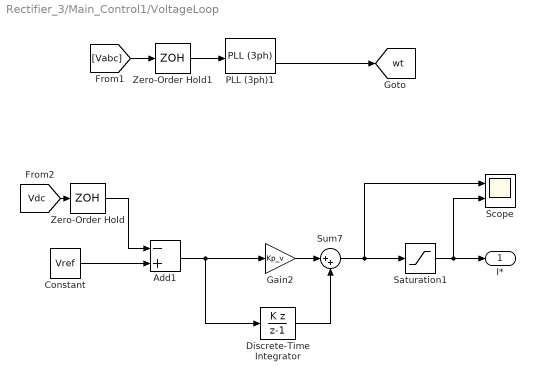
== system Rectifier_3/Main_Control1/VoltageLoop ==
  Add1 : Sum  Inputs=-+
  Constant : Constant  Value=Vref
  Discrete-Time Integrator : DiscreteIntegrator  IntegratorMethod=Accumulation: Backward Euler  gainval=Ki_v  SampleTime=1/Fs/2  ICPrevOutput=DiscIntNeverNeededParam  ICPrevScaledInput=DiscIntNeverNeededParam
  Gain2 : Gain  Gain=Kp_v
  PLL (3ph)1 : spsPLL3phLib/PLL (3ph)  Fmin=45  Par_Init=[0, 60]  ParK=[180, 3200, 1]  TcD=1e-4  MaxRateChangeFreq=12  FilterCutOffFreq=25  Ts=0  AGC=on
  Saturation1 : Saturate  UpperLimit=limit1  LowerLimit=-limit1  SampleTime=1/Fs/2
  Scope : Scope  NumInputPorts=2
  Sum7 : Sum  Inputs=|++
  Zero-Order Hold : ZeroOrderHold  SampleTime=1/Fs/2
  Zero-Order Hold1 : ZeroOrderHold  SampleTime=1/Fs/2
  I* : Outport
  tag scope: wt=global
  wires:
  [Vdc] -> Zero-Order Hold/1
  Zero-Order Hold/1 -> Add1/1
  Constant/1 -> Add1/2
  Saturation1/1 -> I*/1, Scope/2
  Add1/1 -> Discrete-Time Integrator/1, Gain2/1
  Gain2/1 -> Sum7/1
  Discrete-Time Integrator/1 -> Sum7/2
  Sum7/1 -> Scope/1, Saturation1/1
  [Vabc] -> Zero-Order Hold1/1
  Zero-Order Hold1/1 -> PLL (3ph)1/1
  PLL (3ph)1/2 -> [wt]

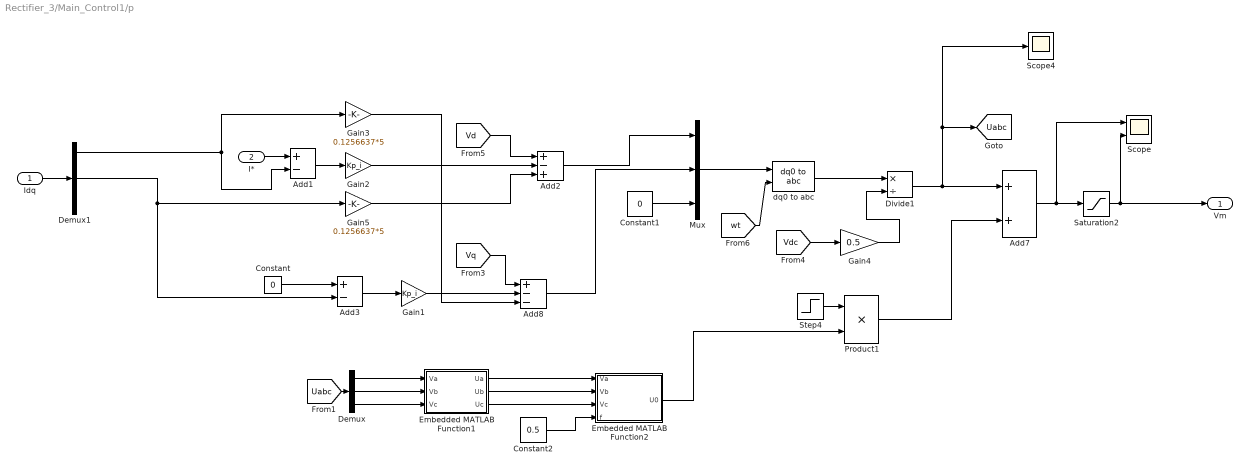
== system Rectifier_3/Main_Control1/p ==
  Idq : Inport
  I* : Inport  Port=2
  Add1 : Sum  Inputs=+-
  Add2 : Sum  Inputs=+-+
  Add3 : Sum  Inputs=+-
  Add7 : Sum
  Add8 : Sum  Inputs=+--
  Constant : Constant  Value=0
  Constant1 : Constant  Value=0
  Constant2 : Constant  Value=0.5
  Demux : Demux  Outputs=3
  Demux1 : Demux  Outputs=3
  Divide1 : Product  Inputs=*/
  Embedded MATLAB Function1 : MATLAB Function  TreatAsAtomicUnit=on
  Embedded MATLAB Function2 : MATLAB Function  TreatAsAtomicUnit=on
  Gain1 : Gain  Gain=Kp_i  SampleTime=1/Fs/2
  Gain2 : Gain  Gain=Kp_i  SampleTime=1/Fs/2
  Gain3 : Gain  Gain=0.1256637*5  SampleTime=1/Fs/2
  Gain4 : Gain  Gain=0.5  SampleTime=1/Fs/2
  Gain5 : Gain  Gain=0.1256637*5  SampleTime=1/Fs/2
  Mux : Mux  Inputs=3
  Product1 : Product
  Saturation2 : Saturate  UpperLimit=1  LowerLimit=-1  SampleTime=1/Fs/2
  Scope : Scope  NumInputPorts=2
  Scope4 : Scope
  Step4 : Step  Time=0.2  SampleTime=0
  dq0 to abc : spsdq0toabcLib/dq0 to abc  Alignment=90 degrees behind phase A axis
  Vm : Outport
  tag scope: Uabc=global
  wires:
  Idq/1 -> Demux1/1
  Gain3/1 -> Add8/3
  Add3/1 -> Gain1/1
  Add1/1 -> Gain2/1
  [Vq] -> Add8/1
  Gain5/1 -> Add2/3
  [Vd] -> Add2/1
  Add8/1 -> Mux/2
  Mux/1 -> dq0 to abc/1
  Constant1/1 -> Mux/3
  Add2/1 -> Mux/1
  [Vdc] -> Gain4/1
  Saturation2/1 -> Vm/1, Scope/2
  Add7/1 -> Scope/1, Saturation2/1
  Demux1/2 -> Add3/2, Gain5/1
  Demux1/1 -> Gain3/1, Add1/2
  Gain2/1 -> Add2/2
  Gain1/1 -> Add8/2
  Gain4/1 -> Divide1/2
  Divide1/1 -> [Uabc], Scope4/1, Add7/1
  Step4/1 -> Product1/1
  Embedded MATLAB Function2/1(U0) -> Product1/2
  [Uabc] -> Demux/1
  Embedded MATLAB Function1/2(Ub) -> Embedded MATLAB Function2/2(Vb)
  Demux/3 -> Embedded MATLAB Function1/3(Vc)
  Demux/2 -> Embedded MATLAB Function1/2(Vb)
  Demux/1 -> Embedded MATLAB Function1/1(Va)
  Embedded MATLAB Function1/1(Ua) -> Embedded MATLAB Function2/1(Va)
  Embedded MATLAB Function1/3(Uc) -> Embedded MATLAB Function2/3(Vc)
  Constant2/1 -> Embedded MATLAB Function2/4(f)
  [wt] -> dq0 to abc/2
  dq0 to abc/1 -> Divide1/1
  Constant/1 -> Add3/1
  I*/1 -> Add1/1
  Product1/1 -> Add7/2

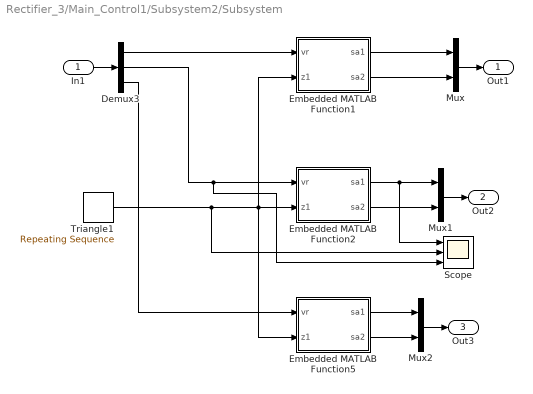
== system Rectifier_3/Main_Control1/Subsystem2/Subsystem ==
  In1 : Inport
  Demux3 : Demux  Outputs=3
  Embedded MATLAB Function1 : MATLAB Function  TreatAsAtomicUnit=on
  Embedded MATLAB Function2 : MATLAB Function  TreatAsAtomicUnit=on
  Embedded MATLAB Function5 : MATLAB Function  TreatAsAtomicUnit=on
  Mux : Mux  Inputs=2
  Mux1 : Mux  Inputs=2
  Mux2 : Mux  Inputs=2
  Scope : Scope  NumInputPorts=3
  Triangle1 : simulink/Sources/Repeating Sequence  rep_seq_t=[0 0.5/Fs 1/Fs]  rep_seq_y=[0 1 0]
  Out1 : Outport
  Out2 : Outport  Port=2
  Out3 : Outport  Port=3
  wires:
  Triangle1/1 -> Scope/2, Embedded MATLAB Function1/2(z1), Embedded MATLAB Function2/2(z1), Embedded MATLAB Function5/2(z1)
  Demux3/1 -> Embedded MATLAB Function1/1(vr)
  Demux3/2 -> Scope/3, Embedded MATLAB Function2/1(vr)
  Demux3/3 -> Embedded MATLAB Function5/1(vr)
  Embedded MATLAB Function1/1(sa1) -> Mux/1
  Embedded MATLAB Function1/2(sa2) -> Mux/2
  Embedded MATLAB Function2/1(sa1) -> Scope/1, Mux1/1
  Embedded MATLAB Function2/2(sa2) -> Mux1/2
  Embedded MATLAB Function5/1(sa1) -> Mux2/1
  Embedded MATLAB Function5/2(sa2) -> Mux2/2
  In1/1 -> Demux3/1
  Mux/1 -> Out1/1
  Mux1/1 -> Out2/1
  Mux2/1 -> Out3/1

== matlab function Rectifier_3/Main_Control1/Subsystem2/Subsystem/Embedded MATLAB Function1 ==
  data: vr input; sa1 output; z1 input; sa2 output
function [sa1,sa2] = PDWM(vr,z1)
% This block supports the Embedded MATLAB subset.
% See the help menu for details.
% Initial for persistent variable
if(vr>0) %zhengbanzhouqi 
    if(vr>z1)
        sa1=0;sa2=1;
    else
        sa1=1;sa2=1;
    end
else     %fubanzhouqi
    vr=vr+1;
    if(vr>z1)
        sa1=1;sa2=1;
    else
        sa1=1;sa2=0;
    end
end

== matlab function Rectifier_3/Main_Control1/Subsystem2/Subsystem/Embedded MATLAB Function2 ==
  data: vr input; sa1 output; z1 input; sa2 output
function [sa1,sa2] = PDWM(vr,z1)
% This block supports the Embedded MATLAB subset.
% See the help menu for details.
% Initial for persistent variable
if(vr>0) %zhengbanzhouqi 
    if(vr>z1)
        sa1=0;sa2=1;
    else
        sa1=1;sa2=1;
    end
else     %fubanzhouqi
    vr=vr+1;
    if(vr>z1)
        sa1=1;sa2=1;
    else
        sa1=1;sa2=0;
    end
end

== matlab function Rectifier_3/Main_Control1/Subsystem2/Subsystem/Embedded MATLAB Function5 ==
  data: vr input; sa1 output; z1 input; sa2 output
function [sa1,sa2] = PDWM(vr,z1)
% This block supports the Embedded MATLAB subset.
% See the help menu for details.
% Initial for persistent variable
if(vr>0) %zhengbanzhouqi 
    if(vr>z1)
        sa1=0;sa2=1;
    else
        sa1=1;sa2=1;
    end
else     %fubanzhouqi
    vr=vr+1;
    if(vr>z1)
        sa1=1;sa2=1;
    else
        sa1=1;sa2=0;
    end
end

== matlab function Rectifier_3/Main_Control1/p/Embedded MATLAB Function1 ==
  data: Va input; Ua output; Vb input; Ub output; Vc input; Uc output
function [Ua,Ub,Uc] = fcn(Va,Vb,Vc)

if Va>=0;
    Ua=Va;
else
    Ua=Va+1;
end
if Vb>=0;
    Ub=Vb;
else
    Ub=Vb+1;
end
if Vc>=0;
    Uc=Vc;
else
    Uc=Vc+1;
end

== matlab function Rectifier_3/Main_Control1/p/Embedded MATLAB Function2 ==
  data: Va input; U0 output; Vb input; Vc input; f input
function U0  = fcn(Va,Vb,Vc,f)

Vmax=Va;         
Vmin=Va;
if Va>=Vb
    Vmin=Vb;
else
    Vmax=Vb;
end
if Vc>=Vmax
    Vmax=Vc;
else 
end
if Vc<=Vmin
    Vmin=Vc;
else
end
U0=f*(1-Vmax+Vmin)-Vmin;
end
